simulink model "plus_generator_edge_trigger"  (R2018a)
settings: Solver=VariableStepAuto  StartTime=0.0  StopTime=10.0  RelTol=1e-3
settings Model: Creator=86188  LastModifiedBy=86188

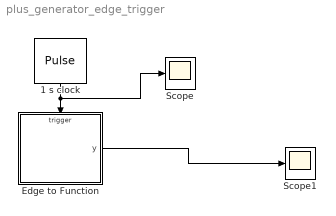
== system plus_generator_edge_trigger ==
  1 s clock : DiscretePulseGenerator  SampleTime=2
  "Edge to Function " : Stateflow chart  TreatAsAtomicUnit=on
  Scope : Scope
  Scope1 : Scope
  wires:
  1 s clock/1 -> Scope/1, "Edge to Function "/Trigger
  "Edge to Function "/1(y) -> Scope1/1

== stateflow chart plus_generator_edge_trigger/Edge to Function  ==
  (default) -> (junction 2) : {y=y+1;}
  data: y output int32 =0
  events: edge input RISING_EDGE_EVENT
